simulink model "Practise2"  (R2017b)
settings: Solver=VariableStepAuto  StartTime=0.0  StopTime=0.05  MaxStep=0.0001  MinStep=0.000099  RelTol=1e-3
values from neighbouring files (symbols this model uses):
  C = 10^4    (= 10000)    [Pracise2.m]
  J1 = 0.046    [Pracise2.m]
  J2 = C*T^2*J1/(J1-C*T^2)    [Pracise2.m]
  mu = ksi*2*T*C    [Pracise2.m]
libraries: fl_lib x7, nesl_utility x3
settings Model: Creator=Aleksandr  LastModifiedBy=Aleksandr

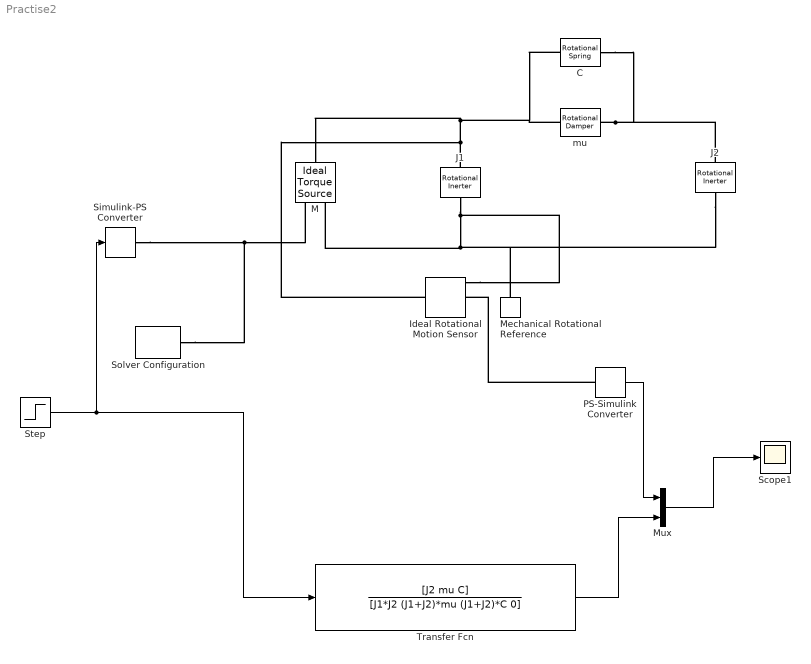
== system Practise2 ==
  C : fl_lib/Mechanical/Rotational Elements/Rotational Spring  spr_rate=C N*m/rad  w_specify=off  w_priority=None  w=0 rad/s  w_nominal_specify=off  w_nominal_unit=rad/s  w_nominal_value=1  t_specify=off  t_priority=None  t=0 N*m  t_nominal_specify=off  t_nominal_unit=N*m  t_nominal_value=1  phi_specify=off  phi_priority=High  phi=0 rad  phi_nominal_specify=off  phi_nominal_unit=rad  phi_nominal_value=1
      settings: SourceProductName=Simscape
  Ideal Rotational Motion Sensor : fl_lib/Mechanical/Mechanical Sensors/Ideal Rotational Motion Sensor  offset=0 rad
  J1 : fl_lib/Mechanical/Rotational Elements/Rotational Inerter  B=J1 kg*m^2  w_specify=off  w_priority=High  w=0 rad/s  w_nominal_specify=off  w_nominal_unit=rad/s  w_nominal_value=1  t_specify=off  t_priority=None  t=0 N*m  t_nominal_specify=off  t_nominal_unit=N*m  t_nominal_value=1
      settings: SourceProductName=Simscape  SourceProductBaseCode=SS
  J2 : fl_lib/Mechanical/Rotational Elements/Rotational Inerter  B=J2 kg*m^2  w_specify=off  w_priority=High  w=0 rad/s  w_nominal_specify=off  w_nominal_unit=rad/s  w_nominal_value=1  t_specify=off  t_priority=None  t=0 N*m  t_nominal_specify=off  t_nominal_unit=N*m  t_nominal_value=1
      settings: SourceProductName=Simscape  SourceProductBaseCode=SS
  M : fl_lib/Mechanical/Mechanical Sources/Ideal Torque Source
  Mechanical Rotational Reference : fl_lib/Mechanical/Rotational Elements/Mechanical Rotational Reference
  Mux : Mux  Inputs=2
  PS-Simulink Converter : nesl_utility/PS-Simulink Converter  PhysicalDomain=network_engine_domain  SubClassName=ps_output  LeftPortType=input  RightPortType=output  PseudoPeriodic=off  Frequencies=[]  Unit=1  AffineConversion=off
  Scope1 : Scope
  Simulink-PS Converter : nesl_utility/Simulink-PS Converter  PhysicalDomain=network_engine_domain  SubClassName=ps_input  LeftPortType=input  RightPortType=output  PseudoPeriodic=off  Frequencies=[]  NoiseDistribution=none  NoiseParameters=[]  Unit=1  AffineConversion=off  FilteringAndDerivatives=provide  SimscapeFilterOrder=1  InputFilterTimeConstant=0.001  UdotUserProvided=0
  Solver Configuration : nesl_utility/Solver Configuration  PhysicalDomain=network_engine_domain  SubClassName=solver  LeftPortType=input  RightPortType=generic  Accelerate=off  Tones=[]  Harmonics=[]  SimulateNoise=off  Profile=off  UseLocalSampling=off  EnableSwitchedLinearOptims=on  FrequencyDomain=off  UseCCode=off  RelTol=0.001  AbsTol=1e-06  MinStep=1e-09  ToWorkspace=off  RevertToSquareIcSolve=off  NumHomotopyIterations=100  PhasorMode=off  PhasorModeNumHarmonics=1  DoDC=off  ResidualTolerance=1e-09  UseLocalSolver=off  LocalSolverChoice=NE_BACKWARD_EULER_ADVANCER  LocalSolverSampleTime=0.001  DoFixedCost=off  MaxNonlinIter=3  MaxModeIter=2  LinearAlgebra=Sparse  DelaysMemoryBudget=1024  AutomaticFiltering=on  FilteringTimeConstant=0.001
  Step : Step  Time=0.05  Before=2  After=0  SampleTime=0
  Transfer Fcn : TransferFcn  Numerator=[J2 mu C]  Denominator=[J1*J2 (J1+J2)*mu (J1+J2)*C 0]
  mu : fl_lib/Mechanical/Rotational Elements/Rotational Damper  D=mu N*m/(rad/s)  w_specify=off  w_priority=None  w=0 rad/s  w_nominal_specify=off  w_nominal_unit=rad/s  w_nominal_value=1  t_specify=off  t_priority=None  t=0 N*m  t_nominal_specify=off  t_nominal_unit=N*m  t_nominal_value=1
  wires:
  Step/1 -> Simulink-PS Converter/1, Transfer Fcn/1
  Mux/1 -> Scope1/1
  PS-Simulink Converter/1 -> Mux/1
  Transfer Fcn/1 -> Mux/2
  connections:
  Simulink-PS Converter/RConn1 -- Solver Configuration/RConn1 -- M/RConn1
  J1/LConn1 -- Ideal Rotational Motion Sensor/LConn1 -- C/LConn1 -- mu/LConn1 -- M/LConn1
  J1/RConn1 -- Ideal Rotational Motion Sensor/RConn1 -- Mechanical Rotational Reference/LConn1 -- J2/RConn1 -- M/RConn2
  mu/RConn1 -- C/RConn1 -- J2/LConn1
  PS-Simulink Converter/LConn1 -- Ideal Rotational Motion Sensor/RConn2
